simulink model "Maglev"  (R2021a)
settings: Solver=VariableStepAuto  StartTime=0.0  StopTime=10.0  RelTol=1e-3
settings Model: Creator=user  LastModifiedBy=user

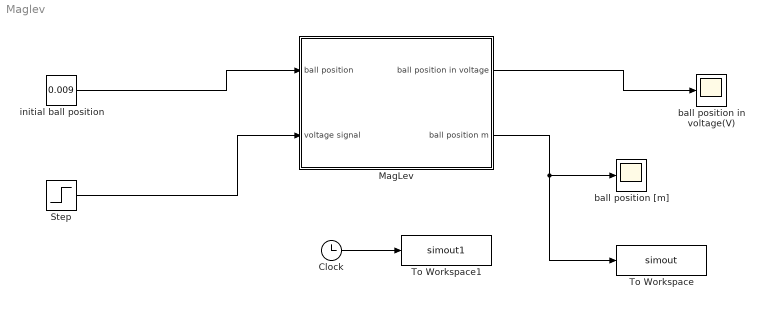
== system Maglev ==
  Clock : Clock
  MagLev : Subsystem
  Step : Step  SampleTime=0
  To Workspace : ToWorkspace  VariableName=simout  SampleTime=0.01
      settings: Save2DSignal=2-D array (concatenate along first dimension)
  To Workspace1 : ToWorkspace  VariableName=simout1  SaveFormat=Timeseries  SampleTime=-1
  ball position [m] : Scope
  ball position in voltage(V) : Scope
  initial ball position : Constant  Value=0.009
  wires:
  initial ball position/1 -> MagLev/1(" ball position")
  Step/1 -> MagLev/2(voltage signal)
  MagLev/2(ball position m) -> To Workspace/1, ball position [m]/1
  Clock/1 -> To Workspace1/1
  MagLev/1(ball position in voltage) -> ball position in voltage(V)/1

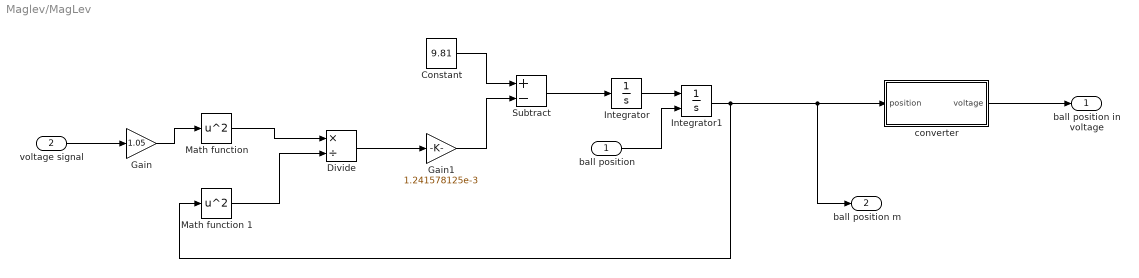
== system Maglev/MagLev ==
  " ball position" : Inport
  voltage signal : Inport  Port=2  Unit=V
  Constant : Constant  Value=9.81
  Divide : Product  Inputs=*/
  Gain : Gain  Gain=1.05
  Gain1 : Gain  Gain=1.241578125e-3
  Integrator : Integrator
  Integrator1 : Integrator  InitialConditionSource=external
  "Math function " : Math  Operator=square  SaturateOnIntegerOverflow=on
  Math function 1 : Math  Operator=square  SaturateOnIntegerOverflow=on
  Subtract : Sum  Inputs=+-
  converter : Subsystem
  ball position in voltage : Outport
  ball position m : Outport  Port=2
  wires:
  voltage signal/1 -> Gain/1
  Gain/1 -> "Math function "/1
  "Math function "/1 -> Divide/1
  Math function 1/1 -> Divide/2
  Divide/1 -> Gain1/1
  Gain1/1 -> Subtract/2
  Constant/1 -> Subtract/1
  Subtract/1 -> Integrator/1
  Integrator/1 -> Integrator1/1
  " ball position"/1 -> Integrator1/2
  Integrator1/1 -> Math function 1/1, ball position m/1, converter/1(position)
  converter/1(voltage) -> ball position in voltage/1

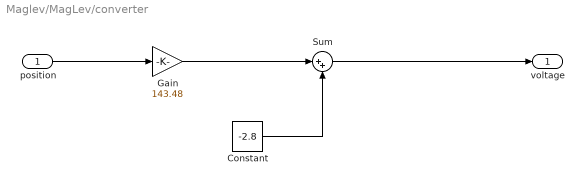
== system Maglev/MagLev/converter ==
  position : Inport
  Constant : Constant  Value=-2.8
  Gain : Gain  Gain=143.48
  Sum : Sum  Inputs=|++
  voltage : Outport
  wires:
  Sum/1 -> voltage/1
  Constant/1 -> Sum/2
  Gain/1 -> Sum/1
  position/1 -> Gain/1
